simulink model "lab_3_qpsk_viterbi"  (R2012b)
settings: Solver=ode45  SolverMode=SingleTasking  StartTime=0.0  StopTime=0.00015  RelTol=1e-3
values from neighbouring files (symbols this model uses):
  EbNodB = 6.4    [lab_3_Pber.m]    (also in lab_3_parameters.m)
  Rb = Nvar*64000    (= 896000)    [lab_3_parameters.m]
  Tb = 1/Rb    (= 1.11607142857e-06)    [lab_3_parameters.m]
undefined symbols (not defined in the file or in its folder): figposition, Fs, sided, Two
libraries: commsink2 x4, dspsigops x2, commcnvcod2 x2, commdigbbndpm3 x2, dspsnks4 x2, commchan3 x1, commrandsrc2 x1, dspindex x1
CloseFcn:
  | clear convSigsOut
settings Model: RequirementInfo=9  CovMetricSettings=d  ExtModeTrigMode=oneshot  ExtModeArmWhenConnect=off  Creator=mikem  LastModifiedBy=yuw
settings DataIOCC: LimitDataPoints=off  SaveOutput=off  SaveTime=off  SignalLoggingName=convSigsOut
settings OptimizationCC: BlockReduction=off  BooleanDataType=off  InitFltsAndDblsToZero=on
settings DebuggingCC: SaveWithParameterizedLinksMsg=none  SignalResolutionControl=TryResolveAllWithWarning  SolverPrmCheckMsg=none  MultiTaskDSMMsg=warning  MultiTaskCondExecSysMsg=none  IntegerOverflowMsg=none  StrictBusMsg=None
settings HardwareCC: TargetUnknown=on
settings RTWCC: IncludeERTFirstTime=on
settings GRTTargetCC: TargetFcnLib=ansi_tfl_tmw.mat  CombineOutputUpdateFcns=off  GRTInterface=on

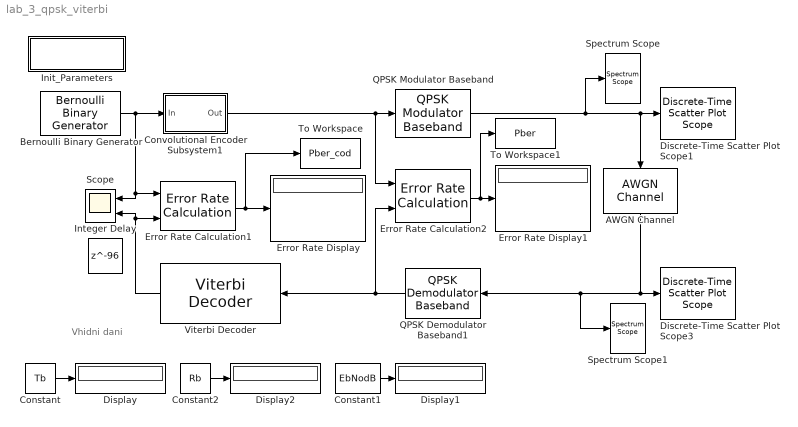
== system lab_3_qpsk_viterbi ==
  note: Vhidni dani
  AWGN Channel : commchan3/AWGN Channel  InputProcessing=Inherited (this choice will be removed - see release notes)  seed=54321  noiseMode="Signal to noise ratio  (Es/No)"  EbNodB=5  EsNodB=EbNodB+10*log10(1/2)  SNRdB=5  bitsPerSym=2  Ps=1  Tsym=1*Tb  variance=1
  Bernoulli Binary Generator : commrandsrc2/Bernoulli Binary Generator  P=0.5  seed=12345  Ts=Tb  frameBased=on  sampPerFrame=1  orient=off  outDataType=double
  Constant : Constant  Value=Tb
  Constant1 : Constant  Value=EbNodB
  Constant2 : Constant  Value=Rb
  Convolutional Encoder Subsystem1 : Subsystem
  Discrete-Time Scatter Plot Scope1 : commsink2/Discrete-Time Scatter Plot Scope  Tag=ScatterPlot  sampPerSymb=1  offsetEye=0  numTraces=40  numNewFrames=10  LineMarkers=.  LineColors=b  fading=on  render=on  AxisGrid=on  xMin=-1.5  xMax=1.5  yMin=-1.5  yMax=1.5  inphaseLabel=In-phase Amplitude  quadratureLabel=Quadrature Amplitude  openScopeAtSimStart=off  FrameNumber=off  FigPos=[360 138 560 560]  figTitle=Scatter Plot  numLinesMax=8  block_type_=scatter
  Discrete-Time Scatter Plot Scope3 : commsink2/Discrete-Time Scatter Plot Scope  Tag=ScatterPlot  sampPerSymb=1  offsetEye=0  numTraces=40  numNewFrames=10  LineMarkers=.  LineColors=b  fading=on  render=on  AxisGrid=on  xMin=-1.5  xMax=1.5  yMin=-1.5  yMax=1.5  inphaseLabel=In-phase Amplitude  quadratureLabel=Quadrature Amplitude  openScopeAtSimStart=off  FrameNumber=off  FigPos=[360 138 560 560]  figTitle=Scatter Plot  numLinesMax=8  block_type_=scatter
  Display : Display
  Display1 : Display
  Display2 : Display
  Error Rate Calculation1 : commsink2/Error Rate Calculation  N=96  st_delay=0  cp_mode=Entire frame  subframe=[]  PMode=Port  WsName=ErrorVec  RsMode2=off  stop=off  numErr=100  maxBits=1e7
  Error Rate Calculation2 : commsink2/Error Rate Calculation  N=0  st_delay=0  cp_mode=Entire frame  subframe=[]  PMode=Port  WsName=ErrorVec  RsMode2=off  stop=off  numErr=100  maxBits=1e6
  Error Rate Display : Display
  Error Rate Display1 : Display
  Init_Parameters : Subsystem
      settings: OpenFcn=lab_3_parameters
      mask Display: disp('lab_3_parameters')
  Integer Delay : Delay  DelayLength=96  InputProcessing=Inherited
  QPSK Demodulator Baseband1 : commdigbbndpm3/QPSK Demodulator Baseband  Ph=pi/4  Dec=Gray  OutType=Integer  DecType=Hard decision  VarSource=Dialog  Variance=1  outDtype1=Inherit via internal rule  outDtype2=Inherit via internal rule  derotateFactorWordLen=16
  QPSK Modulator Baseband : commdigbbndpm3/QPSK Modulator Baseband  InType=Integer  Enc=Gray  Ph=pi/4  outDtype=double  outWordLen=16  outUDDataType=sfix(16)  outFracLenMode=Best precision  outFracLen=15
  Scope : Scope  NumInputPorts=2
      settings: YMin=-2~-2  YMax=2~2
  Spectrum Scope : dspsnks4/Spectrum Scope  ScopeProperties=on  Domain=Frequency  HorizSpan=1  UseBuffer=on  BufferSize=256  Overlap=0  TreatMby1Signals=M channels  inpFftLenInherit=off  FFTlength=128  numAvg=20  DisplayProperties=off  AxisGrid=on  Memory=off  FrameNumber=off  AxisLegend=off  AxisZoom=off  OpenScopeAtSimStart=on  OpenScopeImmediately=off  FigPos="figposition([7    12    39    27])"  AxisProperties=off  XUnits=Hertz  XRange=Two-sided ((-Fs/2...Fs/2])  XDisplay=0  InheritXIncr=on  XIncr=1.0  XLabel=Samples  XLimit=Auto  YUnits=dBW/Hertz  XMax=1  XMin=0  YLabel=Magnitude-squared, dB  LineProperties=off  LineColors=[1 0 0]  wintypeSpecScope=Hann  RsSpecScope=50  betaSpecScope=5  winsampSpecScope=Periodic  XAxisParamsVer=6.8  isFrameUpgraded=on
      settings: YMin=-50  YMax=10
  Spectrum Scope1 : dspsnks4/Spectrum Scope  ScopeProperties=on  Domain=Frequency  HorizSpan=1  UseBuffer=on  BufferSize=256  Overlap=0  TreatMby1Signals=M channels  inpFftLenInherit=off  FFTlength=128  numAvg=20  DisplayProperties=off  AxisGrid=on  Memory=off  FrameNumber=off  AxisLegend=off  AxisZoom=off  OpenScopeAtSimStart=off  OpenScopeImmediately=off  FigPos="figposition([49    12    39    27])"  AxisProperties=off  XUnits=Hertz  XRange=[-Fs/2...Fs/2]  XDisplay=0  InheritXIncr=on  XIncr=1.0  XLabel=Samples  XLimit=Auto  YUnits=dB  XMax=1  XMin=0  YLabel=Magnitude-squared, dB  LineProperties=off  LineColors=[1 0 0]  wintypeSpecScope=Hann  RsSpecScope=50  betaSpecScope=5  winsampSpecScope=Periodic  XAxisParamsVer=6.8  isFrameUpgraded=on
      settings: YMin=-10  YMax=10
  To Workspace : ToWorkspace  VariableName=Pber_cod  SampleTime=-1
      settings: MaxDataPoints=1
  To Workspace1 : ToWorkspace  VariableName=Pber  SampleTime=-1
      settings: MaxDataPoints=1
  Viterbi Decoder : commcnvcod2/Viterbi Decoder  trellis=poly2trellis(7, [171 133])  isPunctured=off  punctureVector=[1; 1; 0; 1; 0; 1]  erasures=off  dectype=Hard decision  runSigValErrCheck=off  nsdecb=4  smWordLength=16  tbdepth=96  opmode=Continuous  reset=off  outDataType=double  delayedResetAction=off
  wires:
  Error Rate Calculation1/1 -> To Workspace/1, Error Rate Display/1
  Convolutional Encoder Subsystem1/1(Out) -> QPSK Modulator Baseband/1, Error Rate Calculation2/1
  QPSK Demodulator Baseband1/1 -> Error Rate Calculation2/2, Viterbi Decoder/1
  Bernoulli Binary Generator/1 -> Error Rate Calculation1/1, Scope/1, Convolutional Encoder Subsystem1/1(In)
  Constant/1 -> Display/1
  Constant1/1 -> Display1/1
  Constant2/1 -> Display2/1
  Error Rate Calculation2/1 -> Error Rate Display1/1, To Workspace1/1
  AWGN Channel/1 -> Spectrum Scope1/1, QPSK Demodulator Baseband1/1, Discrete-Time Scatter Plot Scope3/1
  QPSK Modulator Baseband/1 -> Spectrum Scope/1, AWGN Channel/1, Discrete-Time Scatter Plot Scope1/1
  Viterbi Decoder/1 -> Scope/2, Error Rate Calculation1/2

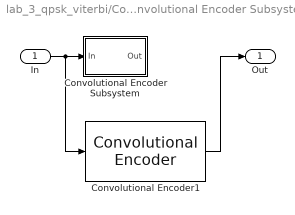
== system lab_3_qpsk_viterbi/Convolutional Encoder Subsystem1 ==
  In : Inport
  Convolutional Encoder Subsystem : Subsystem
  Convolutional Encoder1 : commcnvcod2/Convolutional Encoder  trellis=poly2trellis(7, [171 133])  opMode=Continuous  DelayedResetAction=off  hasIniStPort=off  hasFinStPort=off  usePuncVector=off  punctureVector=[1; 1; 0; 1; 0; 1]  reset=Unused parameter value
  Out : Outport
  wires:
  In/1 -> Convolutional Encoder Subsystem/1(In), Convolutional Encoder1/1
  Convolutional Encoder1/1 -> Out/1

== system lab_3_qpsk_viterbi/Init_Parameters ==

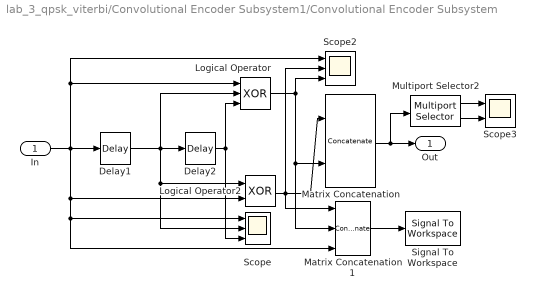
== system lab_3_qpsk_viterbi/Convolutional Encoder Subsystem1/Convolutional Encoder Subsystem ==
  In : Inport
  Delay1 : dspsigops/Delay  InputProcessing=Inherited (this choice will be removed - see release notes)  dly_unit=Samples  delay=1  ic_detail=off  dif_ic_for_ch=off  dif_ic_for_dly=off  ic=0  reset_popup=None
  Delay2 : dspsigops/Delay  InputProcessing=Inherited (this choice will be removed - see release notes)  dly_unit=Samples  delay=1  ic_detail=off  dif_ic_for_ch=off  dif_ic_for_dly=off  ic=0  reset_popup=None
  Logical Operator : Logic  Operator=XOR  Inputs=3  AllPortsSameDT=off
  Logical Operator2 : Logic  Operator=XOR  AllPortsSameDT=off
  Matrix Concatenation : Concatenate  Mode=Multidimensional array
  Matrix Concatenation1 : Concatenate  NumInputs=3  Mode=Multidimensional array  ConcatenateDimension=2
  Multiport Selector2 : dspindex/Multiport Selector  rowsOrCols=Rows  idxCellArray={1 2}  idxErrMode=Clip Index
  Scope : Scope  NumInputPorts=3
      settings: YMin=-5~-5~-5  YMax=5~5~5
  Scope2 : Scope  NumInputPorts=3
      settings: YMin=-5~-5~-5  YMax=5~5~5  SaveName=ScopeData2
  Scope3 : Scope  NumInputPorts=2
      settings: YMin=-5~-5  YMax=5~5  SaveName=ScopeData3
  Signal To Workspace : SignalToWorkspace  VariableName=In_Cod
      settings: CopyFcn=dspblkcopystw(gcbh);
  Out : Outport
  wires:
  Delay2/1 -> Logical Operator/3, Scope/3
  Delay1/1 -> Delay2/1, Logical Operator/2, Scope/2, Logical Operator2/1
  Multiport Selector2/1 -> Scope3/1
  Multiport Selector2/2 -> Scope3/2
  Logical Operator/1 -> Scope2/3, Matrix Concatenation/2, Matrix Concatenation1/2
  Logical Operator2/1 -> Scope2/2, Matrix Concatenation/1, Matrix Concatenation1/1
  In/1 -> Delay1/1, Logical Operator2/2, Scope/1, Matrix Concatenation1/3, Logical Operator/1, Scope2/1
  Matrix Concatenation/1 -> Out/1, Multiport Selector2/1
  Matrix Concatenation1/1 -> Signal To Workspace/1
